simulink library "controller"  (R2020a)
settings: Solver=VariableStepAuto  StartTime=0.0  StopTime=10.0  RelTol=1e-3
undefined symbols (not defined in the file): kd, ki, kp, rDesired, tau
libraries: calculate_vector_magnitude x2, filteredPIDController x2, calcPathCoords x1, findClosestPointOnPath x1, findTargetPathParameter x1, rotationFromGroundToTangent x1
settings Model: Creator=Ayaz  LastModifiedBy=Ayaz

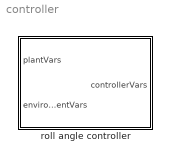
== system controller ==
  roll angle controller : Subsystem  mask{mass=0, pathWidth=0, pathHeight=0, pMeanE=0, Lforward=0, init_s=0, rDes=rDesired, kp=kp, ki=ki, kd=kd, tau=tau}
      mask prompts: mass "Kite mass [kg]"; pathWidth "Path width [deg]"; pathHeight "Path height [deg]"; pMeanE "Path mean elevation angle [deg]"; Lforward "Forward looking length [m]"; init_s "Initial path parameter"; rDes "Desired radius [m]"; kp "Proportional Gain [(m/s)/m]"; ki "Integral Gain [(m/s)/(ms)]"; kd "Derivative Gain [(m/s)/(m/s)]"; tau "Time Constant [s]"
      mask init:
      | w = pathWidth*pi/180;
      | h = pathHeight*pi/180;
      | aBooth = 0.5*w;
      | bBooth = (1/(2*sqrt(2)))*sqrt(-w^2+sqrt((h^2*(4+h^2)*w^4))/(h^2));
      | meanElev = pMeanE*pi/180;
      mask TypeOptions rDes: rDes/Value
      mask TypeOptions kp: filteredPIDController/kp
      mask TypeOptions ki: filteredPIDController/ki
      mask TypeOptions kd: filteredPIDController/kd
      mask TypeOptions tau: filteredPIDController/Value
      mask DialogControl Container4 Prompt: Roll anlge control
      mask DialogControl Container3 Prompt: Spooling control

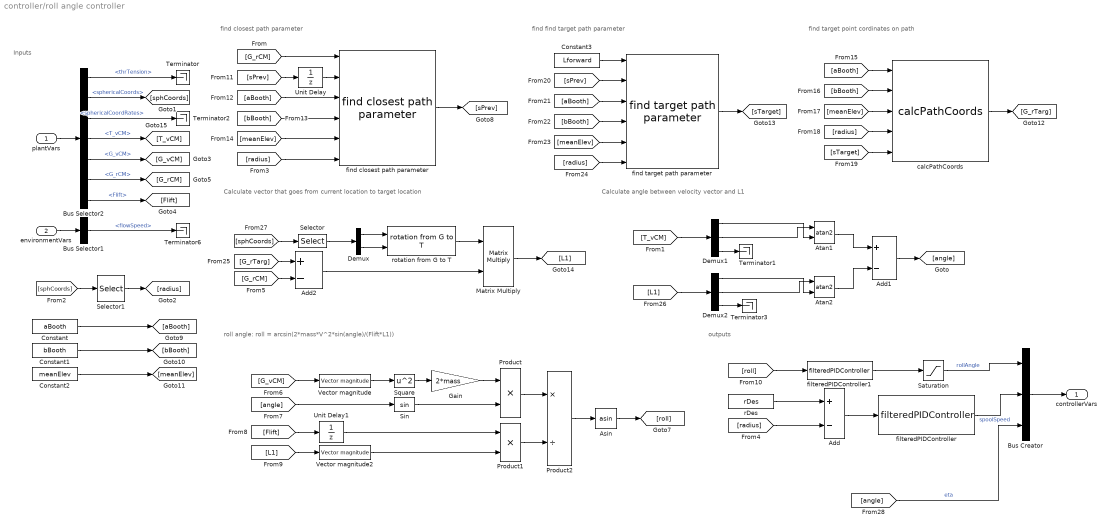
== system controller/roll angle controller ==
  note: Calculate angle between velocity vector and L1
  note: Calculate vector that goes from current location to target location
  note: find closest path parameter
  note: outputs
  note: roll angle: roll = arcsin(2*mass*V^2*sin(angle)/(Flift*L1))
  note: Inputs
  note: find find target path parameter
  note: find target point cordinates on path
  plantVars : Inport
  environmentVars : Inport  Port=2
  Add : Sum  Inputs=+-
  Add1 : Sum  Inputs=+-
  Add2 : Sum  Inputs=+-
  Asin : Trigonometry  Operator=asin
  Atan1 : Trigonometry  Operator=atan2
  Atan2 : Trigonometry  Operator=atan2
  Bus Creator : BusCreator  Inputs=3
  Bus Selector1 : BusSelector  OutputSignals=flowSpeed
  Bus Selector2 : BusSelector  OutputSignals=thrTension,sphericalCoords,sphericalCoordRates,T_vCM,G_vCM,G_rCM,Flift
  Constant : Constant  Value=aBooth
  Constant1 : Constant  Value=bBooth
  Constant2 : Constant  Value=meanElev
  Constant3 : Constant  Value=Lforward  VectorParams1D=off
  Demux : Demux  Outputs=2
  Demux1 : Demux  Outputs=3
  Demux2 : Demux  Outputs=3
  Gain : Gain  Gain=2*mass
  Matrix Multiply : Product  Multiplication=Matrix(*)
  Product : Product
  Product1 : Product
  Product2 : Product  Inputs=*/
  Saturation : Saturate  UpperLimit=90*pi/180  LowerLimit=-90*pi/180
  Selector : Selector  InputPortWidth=3  IndexOptions=Index vector (dialog)  Indices=[1 2]  OutputSizes=1
  Selector1 : Selector  InputPortWidth=3  IndexOptions=Index vector (dialog)  Indices=3  OutputSizes=1
  Sin : Trigonometry
  Square : Math  Operator=square  SaturateOnIntegerOverflow=on
  Terminator{,1..3,6} (5 alike) : Terminator
  Unit Delay : UnitDelay  InitialCondition=init_s  SampleTime=-1  HasFrameUpgradeWarning=on
  Unit Delay1 : UnitDelay  InitialCondition=mass  SampleTime=-1  HasFrameUpgradeWarning=on
  Vector magnitude : calculate_vector_magnitude/Vector magnitude  SystemSampleTime=-1  Latency=0  AutoFrameSizeCalculation=off
  Vector magnitude2 : calculate_vector_magnitude/Vector magnitude  SystemSampleTime=-1  Latency=0  AutoFrameSizeCalculation=off
  calcPathCoords : calcPathCoords/calcPathCoords  SystemSampleTime=-1  Latency=0  AutoFrameSizeCalculation=off
  filteredPIDController : filteredPIDController/filteredPIDController  kp=kp  ki=ki  kd=kd  Value=tau  externalReset=none
  filteredPIDController1 : filteredPIDController/filteredPIDController  kp=1  ki=0  kd=0  Value=0.01  externalReset=none
  find closest path parameter : findClosestPointOnPath/find closest path parameter  SystemSampleTime=-1  Latency=0  AutoFrameSizeCalculation=off
  find target path parameter : findTargetPathParameter/find target path parameter  SystemSampleTime=-1  Latency=0  AutoFrameSizeCalculation=off
  rDes : Constant  Value=rDes
  rotation from G to T : rotationFromGroundToTangent/rotation from G to T  SystemSampleTime=-1  Latency=0  AutoFrameSizeCalculation=off
  controllerVars : Outport
  wires:
  plantVars/1 -> Bus Selector2/1
  Bus Selector2/1 -> Terminator/1  "<thrTension>"
  Bus Selector2/2 -> [sphCoords]  "<sphericalCoords>"
  Bus Selector2/3 -> Terminator2/1  "<sphericalCoordRates>"
  Bus Selector2/4 -> [T_vCM]  "<T_vCM>"
  Bus Selector2/5 -> [G_vCM]  "<G_vCM>"
  Bus Selector2/6 -> [G_rCM]  "<G_rCM>"
  Bus Selector1/1 -> Terminator6/1  "<flowSpeed>"
  environmentVars/1 -> Bus Selector1/1
  Saturation/1 -> Bus Creator/1  "rollAngle"
  filteredPIDController/1 -> Bus Creator/2  "spoolSpeed"
  Bus Creator/1 -> controllerVars/1
  [G_rCM] -> find closest path parameter/1
  Add/1 -> filteredPIDController/1
  Selector1/1 -> [radius]
  [sphCoords] -> Selector1/1
  [radius] -> find closest path parameter/6
  [radius] -> Add/2
  Bus Selector2/7 -> [Flift]  "<Flift>"
  [G_vCM] -> Vector magnitude/1
  Vector magnitude/1 -> Square/1
  Square/1 -> Gain/1
  Gain/1 -> Product/1
  [angle] -> Sin/1
  Sin/1 -> Product/2
  [Flift] -> Unit Delay1/1
  [L1] -> Vector magnitude2/1
  Product/1 -> Product2/1
  Product1/1 -> Product2/2
  Product2/1 -> Asin/1
  Asin/1 -> [roll]
  rDes/1 -> Add/1
  find closest path parameter/1 -> [sPrev]
  [sPrev] -> Unit Delay/1
  Unit Delay/1 -> find closest path parameter/2
  Constant2/1 -> [meanElev]
  Constant/1 -> [aBooth]
  Constant1/1 -> [bBooth]
  [aBooth] -> find closest path parameter/3
  [bBooth] -> find closest path parameter/4
  [meanElev] -> find closest path parameter/5
  [meanElev] -> calcPathCoords/3
  [bBooth] -> calcPathCoords/2
  [aBooth] -> calcPathCoords/1
  [radius] -> calcPathCoords/4
  calcPathCoords/1 -> [G_rTarg]
  [sPrev] -> find target path parameter/2
  [radius] -> find target path parameter/6
  [aBooth] -> find target path parameter/3
  [bBooth] -> find target path parameter/4
  [meanElev] -> find target path parameter/5
  Constant3/1 -> find target path parameter/1
  find target path parameter/1 -> [sTarget]
  [sTarget] -> calcPathCoords/5
  [G_rTarg] -> Add2/1
  [G_rCM] -> Add2/2
  Add2/1 -> Matrix Multiply/2
  Vector magnitude2/1 -> Product1/2
  [T_vCM] -> Demux1/1
  Unit Delay1/1 -> Product1/1
  [roll] -> filteredPIDController1/1
  filteredPIDController1/1 -> Saturation/1
  [sphCoords] -> Selector/1
  Selector/1 -> Demux/1
  Demux/1 -> rotation from G to T/1
  Demux/2 -> rotation from G to T/2
  rotation from G to T/1 -> Matrix Multiply/1
  Matrix Multiply/1 -> [L1]
  Demux1/3 -> Terminator1/1
  Demux1/1 -> Atan1/2
  Demux1/2 -> Atan1/1
  Demux2/3 -> Terminator3/1
  [L1] -> Demux2/1
  Demux2/2 -> Atan2/1
  Demux2/1 -> Atan2/2
  Atan1/1 -> Add1/1
  Atan2/1 -> Add1/2
  Add1/1 -> [angle]
  [angle] -> Bus Creator/3  "eta"
